simulink model "motor_dc_simulink"  (R2021a)
settings: Solver=VariableStepAuto  StartTime=0.0  StopTime=60  RelTol=1e-3
values from neighbouring files (symbols this model uses):
  K = [zeros(1,size(A,1)-1)  1]*inv(Co)*( A^2 + alphacontz(2)*A + alphacontz(3)*eye(size(A)) )    [motor_dc.m]
  Ts = 0.15    [motor_dc.m]
undefined symbols (not defined in the file or in its folder): Ac, Bc, Cc, sigbuilder_block
settings Model: Creator=Dell  LastModifiedBy=Dell
settings SolverCC: AlgebraicLoopSolver=TrustRegion
settings DebuggingCC: SFMachineParentedDataDiag=warning

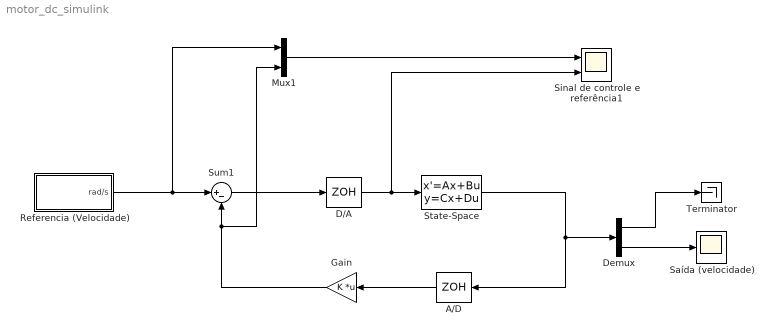
== system motor_dc_simulink ==
  A/D : ZeroOrderHold  SampleTime=Ts
  D/A : ZeroOrderHold  SampleTime=Ts
  Demux : Demux  Outputs=2
  Gain : Gain  Gain=K  Multiplication=Matrix(K*u)
  Mux1 : Mux  Inputs=2
  Referencia (Velocidade) : Subsystem  Tag=STV Subsys  LoadFcn=sigbuilder_block('load');  StartFcn=sigbuilder_block('start');  StopFcn=sigbuilder_block('stop');  ClipboardFcn=sigbuilder_block('clipboard');  mask(Sigbuilder block){tuvar=[0:10]}
      mask help: Sigbuilder GUI
      mask init:
      | if ~strcmp(get_param(bdroot(gcbh),'SimulationStatus'),'stopped') tuvar = sigbuilder_block('maskInit'); end
      settings: CopyFcn=sigbuilder_block('copy');  DeleteFcn=sigbuilder_block('delete');  ModelCloseFcn=sigbuilder_block('modelClose');  PreSaveFcn=sigbuilder_block('preSave');  PauseFcn=sigbuilder_block('pause')  ContinueFcn=sigbuilder_block('continue')  NameChangeFcn=sigbuilder_block('namechange');  OpenFcn=sigbuilder_block('open',[6 30 1012.5 447.75 ]);  CloseFcn=sigbuilder_block('close');
      mask Display: plot(0, 0, 100, 100,[2, 2, 32, 32, 2], [68, 8, 8, 68, 68],[32, 2], [38, 38], [32, 19, 2],[53, 60, 44], [32, 17, 17, 2],[16, 16, 31, 31]);txt = getActiveGroup(gcbh);text(2, 100, txt,'verticalAlignment', 'top');
  Saída (velocidade) : Scope
  Sinal de controle e referência1 : Scope  NumInputPorts=2
  State-Space : StateSpace  A=Ac  B=Bc  C=[1 0; Cc]  D=[0; 0]  InitialCondition=0  ParameterTunability=Optimized
  Sum1 : Sum  Inputs=|+-
  Terminator : Terminator
  wires:
  Gain/1 -> Mux1/2, Sum1/2
  Referencia (Velocidade)/1(rad/s) -> Mux1/1, Sum1/1
  Demux/2 -> Saída (velocidade)/1
  Demux/1 -> Terminator/1
  Sum1/1 -> D/A/1
  D/A/1 -> Sinal de controle e referência1/2, State-Space/1
  A/D/1 -> Gain/1
  Mux1/1 -> Sinal de controle e referência1/1
  State-Space/1 -> Demux/1, A/D/1

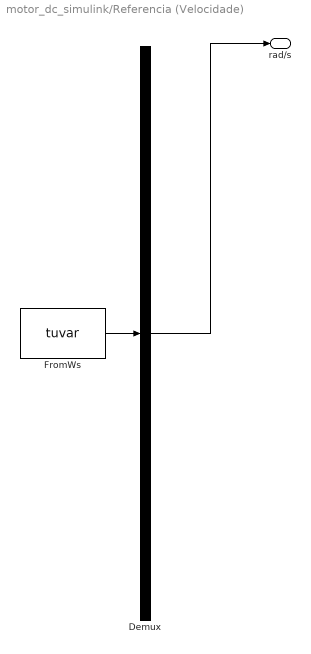
== system motor_dc_simulink/Referencia (Velocidade) ==
  Demux : Demux  Tag=STV Demux  Outputs=1
      settings: DisplayOption=none
  FromWs : FromWorkspace  Tag=STV FromWs  VariableName=tuvar
      SigBuilderData=|
      | common.afterFinalStr = 'Extrapolate'
      | common.sampleTime = 0
      | dataSet.timeRange = [0 60]
      | dataSet.name = 'Group 1'
      | sbobj.Groups.Name = 'Group 1'
      | sbobj.Groups.Signals.Name = 'rad/s'
      | sbobj.Groups.Signals.XData = [0 10 30 40 60]
      | sbobj.Groups.Signals.YData = [0 100 100 75 0]
      | sbobj.Groups.TimeRange = [0 60]
  rad/s : Outport  Tag=STV Outport
  wires:
  FromWs/1 -> Demux/1
  Demux/1 -> rad/s/1
